simulink model "Differential_robot_kinematic_model"  (R2024b)
settings: Solver=VariableStepAuto  StartTime=0.0  StopTime=10.0  RelTol=1e-3
values from neighbouring files (symbols this model uses):
  L = 150e-3    (= 0.15)    [Init_parameters_Dynamic.m]    (also in Init_parameters_kinematic.m)
  r = 25e-3    (= 0.025)    [Init_parameters_Dynamic.m]    (also in Init_parameters_kinematic.m)
  theta = 0    [Init_parameters_Dynamic.m]    (also in Init_parameters_kinematic.m)
  x = 0    [Init_parameters_Dynamic.m]    (also in Init_parameters_kinematic.m)
  y = 0    [Init_parameters_Dynamic.m]    (also in Init_parameters_kinematic.m)
settings Model: Creator=Nabil  LastModifiedBy=Nabil

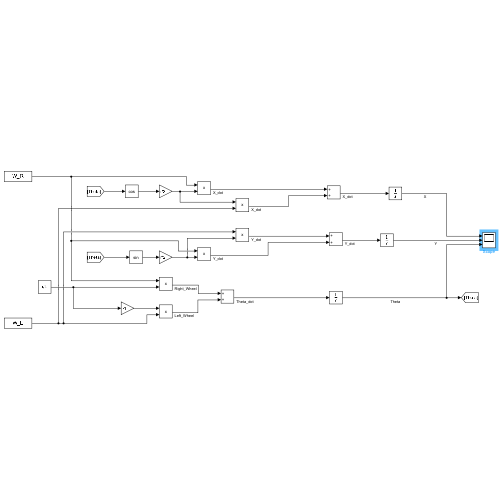
[thumbnail: Simulink's stored preview of the top-level diagram]
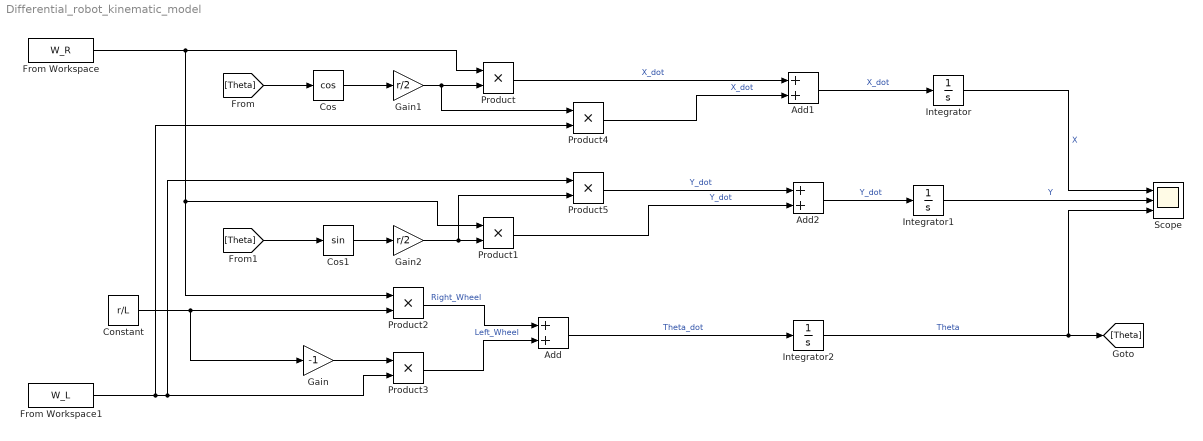
== system Differential_robot_kinematic_model ==
  Add : Sum
  Add1 : Sum
  Add2 : Sum
  Constant : Constant  Value=r/L
  Cos : Trigonometry  Operator=cos
  Cos1 : Trigonometry
  From Workspace : FromWorkspace  VariableName=W_R
  From Workspace1 : FromWorkspace  VariableName=W_L
  Gain : Gain  Gain=-1
  Gain1 : Gain  Gain=r/2
  Gain2 : Gain  Gain=r/2
  Integrator : Integrator  InitialCondition=x
  Integrator1 : Integrator  InitialCondition=y
  Integrator2 : Integrator  InitialCondition=theta
  Product{,1..5} (6 alike) : Product
  Scope : Scope  NumInputPorts=3
  wires:
  Integrator1/1 -> Scope/2  "Y"
  Integrator/1 -> Scope/1  "X"
  Integrator2/1 -> Scope/3, [Theta]  "Theta"
  Cos1/1 -> Gain2/1
  Cos/1 -> Gain1/1
  Add1/1 -> Integrator/1  "X_dot"
  Add2/1 -> Integrator1/1  "Y_dot"
  Add/1 -> Integrator2/1  "Theta_dot"
  Product2/1 -> Add/1  "Right_Wheel"
  Product3/1 -> Add/2  "Left_Wheel"
  [Theta] -> Cos/1
  [Theta] -> Cos1/1
  From Workspace/1 -> Product1/1, Product2/1, Product/1
  From Workspace1/1 -> Product4/2, Product5/1, Product3/2
  Constant/1 -> Gain/1, Product2/2
  Gain/1 -> Product3/1
  Product/1 -> Add1/1  "X_dot"
  Product1/1 -> Add2/2  "Y_dot"
  Product5/1 -> Add2/1  "Y_dot"
  Product4/1 -> Add1/2  "X_dot"
  Gain1/1 -> Product4/1, Product/2
  Gain2/1 -> Product5/2, Product1/2
